simulink model "TLC"  (R2022b)
settings: configuration reference "ERT" (kept outside this file)
undefined symbols (not defined in the file): EGM, FID, IdcMin_P, kiIdcMax_P, kiIdcMin_P, kpIdcMax_P, kpIdcMin_P, OmMechnLimMin_P, pwrIdcMaxDev_P, pwrIdcMinDev_P, SC_fLoLim_C, SC_fUpLim_C, SC_PwrMax_P, SC_TrqMax_P, TQL, trqAddMax_P, trqAddMin_P, Ts_10ms
libraries: simulink x50, MathLib x8, DSMLib x2, slpidlib x1
(part 2 of 2)

== system TLC/TLC_EM/EmOperLim ==
  udclink : Inport
  n : Inport  Port=2
  Abs : Abs  SaturateOnIntegerOverflow=off
  Bus Creator : BusCreator  Inputs=2
  Product : Product
  Product1 : Product
  TrqEmGen_T : Lookup_n-D  DataSpecification=Lookup table object  LookupTableObject=TrqEmGen_T  BreakpointsForDimension1=[250,300,350,400]  BreakpointsForDimension2=[0,500,1000,1500,2000,2500,3000,3500,4000,4500,5000,5500,6000,6500,7000,7500,8000,8500,9000,9500,10000,10500,11000,11500,12000,12500,13000,13500,14000,14500,15000]  BeginIndexSearchUsingPreviousIndexResult=on  Table=reshape([350,350,350,350,350,350,350,350,350,350,350,350,350,350,350,350,350,350,350,350,350,350,350,350,350,350,350,350,350,350,350,350,350,350,350,350,350,350,350,350,350,350,350,350,350,350,350,350,350,350,350,350,350,350,350,350,350,350,350,350,350,350,350,350,350,350,350,350,350,350,350,350,350,350,350,350,350,350,350,350,350,350,350,350,350,350,350,350,350,350,350,350,350,350,350,350,350,350,350,350,350,350,350,350,350,350,350,350,350,350,350,350,350,350,350,350,350,350,350,350,0,0,0,0],4,31)  ExtrapMethod=Clip  UseLastTableValue=on  InternalRulePriority=Speed  OutDataTypeStr=Inherit: Inherit from 'Table data'  RndMeth=Simplest
      settings: InputPortMap=u0,u1
  TrqEmMot_T : Lookup_n-D  DataSpecification=Lookup table object  LookupTableObject=TrqEmMot_T  BreakpointsForDimension1=[250,300,350,400]  BreakpointsForDimension2=[0,500,1000,1500,2000,2500,3000,3500,4000,4500,5000,5500,6000,6500,7000,7500,8000,8500,9000,9500,10000,10500,11000,11500,12000,12500,13000,13500,14000,14500,15000]  BeginIndexSearchUsingPreviousIndexResult=on  Table=reshape([350,350,350,350,350,350,350,350,350,350,350,350,350,350,350,350,350,350,350,350,350,350,350,350,350,350,350,350,350,350,350,350,350,350,350,350,350,350,350,350,350,350,350,350,350,350,350,350,350,350,350,350,350,350,350,350,350,350,350,350,350,350,350,350,350,350,350,350,350,350,350,350,350,350,350,350,350,350,350,350,350,350,350,350,350,350,350,350,350,350,350,350,350,350,350,350,350,350,350,350,350,350,350,350,350,350,350,350,350,350,350,350,350,350,350,350,350,350,350,350,0,0,0,0],4,31)  ExtrapMethod=Clip  UseLastTableValue=on  InternalRulePriority=Speed  OutDataTypeStr=Inherit: Inherit from 'Table data'  RndMeth=Simplest
      settings: InputPortMap=u0,u1
  trqMax : Constant  Value=SC_TrqMax_P  OutDataTypeStr=single
  OperLim : Outport  VectorParamsAs1DForOutWhenUnconnected=off
  wires:
  n/1 -> Abs/1
  Abs/1 -> TrqEmGen_T/2, TrqEmMot_T/2
  TrqEmMot_T/1 -> Product/1
  TrqEmGen_T/1 -> Product1/2
  udclink/1 -> TrqEmGen_T/1, TrqEmMot_T/1
  Bus Creator/1 -> OperLim/1
  Product1/1 -> Bus Creator/2  "trqGenOperLim"
  Product/1 -> Bus Creator/1  "trqMotOperLim"
  trqMax/1 -> Product1/1, Product/2

== system TLC/TLC_EM/IdcLimit ==
  In1 : Inport
  Bus Creator : BusCreator  Inputs=3
  Compare To Constant : simulink/Logic and Bit Operations/Compare To Constant  relop=<  const=1  OutDataTypeStr=boolean
  GLB_PwrMax_P : Constant  Value=SC_TrqMax_P  OutDataTypeStr=single
  Product : Product
  Unary Minus3 : UnaryMinus
  trqGenMotIdcLnkLim_T : Lookup_n-D  NumberOfTableDimensions=1  DataSpecification=Lookup table object  LookupTableObject=trqGenMotIdcLnkLim_T  BreakpointsForDimension1=[-3500 -3000 0 7000 7200]  BeginIndexSearchUsingPreviousIndexResult=on  Table=[0 1 1 1 0]  ExtrapMethod=Clip  UseLastTableValue=on  InternalRulePriority=Speed  OutDataTypeStr=Inherit: Inherit from 'Table data'  RndMeth=Simplest
  IdcLnkLim : Outport  VectorParamsAs1DForOutWhenUnconnected=off
  wires:
  In1/1 -> trqGenMotIdcLnkLim_T/1
  Unary Minus3/1 -> Bus Creator/2  "trqGenIdcLinkLim"
  trqGenMotIdcLnkLim_T/1 -> Compare To Constant/1, Product/2
  Compare To Constant/1 -> Bus Creator/3  "bTrqnLimActv"
  Bus Creator/1 -> IdcLnkLim/1
  GLB_PwrMax_P/1 -> Product/1
  Product/1 -> Bus Creator/1, Unary Minus3/1  "trqMotIdcLinkLim"

== system TLC/TLC_EM/TempClntLim ==
  TempInv : Inport
  Bus Creator : BusCreator  Inputs=3
  GLB_TrqMax_P2 : Constant  Value=SC_TrqMax_P  OutDataTypeStr=single
  Logical Operator : Logic  Operator=OR  AllPortsSameDT=off  OutDataTypeStr=boolean
  Product : Product
  Product1 : Product
  Relational Operator : RelationalOperator  OutDataTypeStr=boolean  RndMeth=Simplest  InputSameDT=off
  Relational Operator1 : RelationalOperator  OutDataTypeStr=boolean  RndMeth=Simplest  InputSameDT=off
  Unary Minus : UnaryMinus
  trqGenTInvLim_T : Lookup_n-D  NumberOfTableDimensions=1  DataSpecification=Lookup table object  LookupTableObject=trqGenTClntLim_T  BreakpointsForDimension1=[100 125 135]  BeginIndexSearchUsingPreviousIndexResult=on  Table=[1 0.8 0]  ExtrapMethod=Clip  UseLastTableValue=on  InternalRulePriority=Speed  OutDataTypeStr=Inherit: Inherit from 'Table data'  RndMeth=Simplest
  trqMotTInvLim_T : Lookup_n-D  NumberOfTableDimensions=1  DataSpecification=Lookup table object  LookupTableObject=trqMotTClntLim_T  BreakpointsForDimension1=[100 125 135]  BeginIndexSearchUsingPreviousIndexResult=on  Table=[1 0.8 0]  ExtrapMethod=Clip  UseLastTableValue=on  InternalRulePriority=Speed  OutDataTypeStr=Inherit: Inherit from 'Table data'  RndMeth=Simplest
  TClntLim : Outport  VectorParamsAs1DForOutWhenUnconnected=off
  wires:
  Product1/1 -> Unary Minus/1, Relational Operator1/2
  trqGenTInvLim_T/1 -> Product1/2
  Unary Minus/1 -> Bus Creator/2  "trqGenTClntLim"
  Bus Creator/1 -> TClntLim/1
  trqMotTInvLim_T/1 -> Product/2
  TempInv/1 -> trqGenTInvLim_T/1, trqMotTInvLim_T/1
  Product/1 -> Bus Creator/1, Relational Operator/2  "trqMotTClntLim"
  GLB_TrqMax_P2/1 -> Relational Operator1/1, Relational Operator/1, Product1/1, Product/1
  Relational Operator/1 -> Logical Operator/1  "bTrqMotTClntLimActv"
  Relational Operator1/1 -> Logical Operator/2  "bTrqGenTClntLimActv"
  Logical Operator/1 -> Bus Creator/3  "bTrqTClntLimActv"

== system TLC/TLC_EM/TempInvLim ==
  TempInv : Inport
  Bus Creator : BusCreator  Inputs=3
  GLB_TrqMax_P2 : Constant  Value=SC_TrqMax_P  OutDataTypeStr=single
  Logical Operator : Logic  Operator=OR  AllPortsSameDT=off  OutDataTypeStr=boolean
  Product : Product
  Product1 : Product
  Relational Operator : RelationalOperator  OutDataTypeStr=boolean  RndMeth=Simplest  InputSameDT=off
  Relational Operator1 : RelationalOperator  OutDataTypeStr=boolean  RndMeth=Simplest  InputSameDT=off
  Unary Minus : UnaryMinus
  trqGenTInvLim_T : Lookup_n-D  NumberOfTableDimensions=1  DataSpecification=Lookup table object  LookupTableObject=trqGenTInvLim_T  BreakpointsForDimension1=[100 125 135]  BeginIndexSearchUsingPreviousIndexResult=on  Table=[1 0.8 0]  ExtrapMethod=Clip  UseLastTableValue=on  InternalRulePriority=Speed  OutDataTypeStr=Inherit: Inherit from 'Table data'  RndMeth=Simplest
  trqMotTInvLim_T : Lookup_n-D  NumberOfTableDimensions=1  DataSpecification=Lookup table object  LookupTableObject=trqMotTInvLim_T  BreakpointsForDimension1=[100 125 135]  BeginIndexSearchUsingPreviousIndexResult=on  Table=[1 0.8 0]  ExtrapMethod=Clip  UseLastTableValue=on  InternalRulePriority=Speed  OutDataTypeStr=Inherit: Inherit from 'Table data'  RndMeth=Simplest
  TInvLim : Outport  VectorParamsAs1DForOutWhenUnconnected=off
  wires:
  Product1/1 -> Unary Minus/1, Relational Operator1/2
  trqGenTInvLim_T/1 -> Product1/2
  Unary Minus/1 -> Bus Creator/2  "trqGenTInvLim"
  Bus Creator/1 -> TInvLim/1
  trqMotTInvLim_T/1 -> Product/2
  TempInv/1 -> trqGenTInvLim_T/1, trqMotTInvLim_T/1
  Product/1 -> Bus Creator/1, Relational Operator/2  "trqMotTInvLim"
  GLB_TrqMax_P2/1 -> Relational Operator1/1, Relational Operator/1, Product1/1, Product/1
  Relational Operator/1 -> Logical Operator/1  "bTrqMotTInvLimActv"
  Relational Operator1/1 -> Logical Operator/2  "bTrqGenTInvLimActv"
  Logical Operator/1 -> Bus Creator/3  "bTrqTinvLimActv"

== system TLC/TLC_EM/TempRtrLim ==
  note: <TODO, change the FID identifier>
  TempRtr : Inport
  Bus Creator1 : BusCreator  Inputs=7
  Bus Creator2 : BusCreator  Inputs=7
  Disable : Subsystem  TreatAsAtomicUnit=on
  Enable : Subsystem  TreatAsAtomicUnit=on
  Enumerated Constant1 : simulink/Sources/Enumerated Constant  OutDataTypeStr=Enum: FID  Value=FID.ReqStandby  SampleTime=inf
      settings: AttributesFormatString=|
      | -------------------------------
      | Enable limitor according to status temperature
  Switch : Switch  Criteria=u2 > Threshold  SaturateOnIntegerOverflow=off  InputSameDT=off
  getFIdSim : DSMLib/getFIdSim  SystemSampleTime=-1  VariantActivationTime=update diagram  Latency=0  AutoFrameSizeCalculation=off
  TRtrLim : Outport  VectorParamsAs1DForOutWhenUnconnected=off
  wires:
  TempRtr/1 -> Disable/1(TmpRtr), Enable/1(TmpRtr)
  Switch/1 -> TRtrLim/1
  Disable/1(pwrMotTRtrLim) -> Bus Creator1/1
  Disable/2(pwrGenTRtrLim) -> Bus Creator1/2
  Disable/3(trqMotTRtrLim) -> Bus Creator1/3
  Disable/4(trqGenTRtrLim) -> Bus Creator1/4
  Disable/5(bTRtrLimActv) -> Bus Creator1/5
  Disable/6(bTrqMotTRtrLimDfcAcive) -> Bus Creator1/6
  Disable/7(bTrqGenTRtrLimDfcAcive) -> Bus Creator1/7
  Enable/1(pwrMotTRtrLim) -> Bus Creator2/1
  Enable/2(pwrGenTRtrLim) -> Bus Creator2/2
  Enable/3(trqMotTRtrLim) -> Bus Creator2/3
  Enable/4(trqGenTRtrLim) -> Bus Creator2/4
  Enable/5(bTRtrLimActv) -> Bus Creator2/5
  Enable/6(bTrqMotTRtrLimDfcAcive) -> Bus Creator2/6
  Enable/7(bTrqGenTRtrLimDfcAcive) -> Bus Creator2/7
  Bus Creator2/1 -> Switch/1
  Bus Creator1/1 -> Switch/3
  Enumerated Constant1/1 -> getFIdSim/1
  getFIdSim/1 -> Switch/2

== system TLC/TLC_EM/TempStrLim ==
  TempStr : Inport
  Bus Creator : BusCreator  Inputs=7
  Enumerated Constant2 : simulink/Sources/Enumerated Constant  OutDataTypeStr=Enum: FID  Value=FID.ReqStandby  SampleTime=inf
      settings: AttributesFormatString=|
      | -------------------------------
      | Enable limitor according to status temperature
  If : If  IfExpression=u1
  If Action Subsystem : Subsystem  TreatAsAtomicUnit=on
  If Action Subsystem1 : Subsystem  TreatAsAtomicUnit=on
  Merge{,1..6} (7 alike) : Merge  InitialOutput=false
  getFIdSim : DSMLib/getFIdSim  SystemSampleTime=-1  VariantActivationTime=update diagram  Latency=0  AutoFrameSizeCalculation=off
  TStrLim : Outport  VectorParamsAs1DForOutWhenUnconnected=off
  wires:
  If/1 -> If Action Subsystem/Action
  If/2 -> If Action Subsystem1/Action
  TempStr/1 -> If Action Subsystem1/1(TmpStr), If Action Subsystem/1(TmpStr)
  If Action Subsystem/1(pwrMotTstrLim) -> Merge/1
  If Action Subsystem/2(pwrGenTstrLim) -> Merge1/1
  If Action Subsystem/7(bTrqGenTstrLimDfcAcive) -> Merge6/1
  If Action Subsystem/6(bTrqMotTstrLimDfcAcive) -> Merge5/1
  If Action Subsystem/5(bTstrLimActv) -> Merge4/1
  If Action Subsystem/4(trqGenTstrLim) -> Merge3/1
  If Action Subsystem/3(trqMotTstrLim) -> Merge2/1
  If Action Subsystem1/1(pwrMotTstrLim) -> Merge/2
  If Action Subsystem1/2(pwrGenTstrLim) -> Merge1/2
  If Action Subsystem1/3(trqMotTstrLim) -> Merge2/2
  If Action Subsystem1/4(trqGenTstrLim) -> Merge3/2
  If Action Subsystem1/5(bTstrLimActv) -> Merge4/2
  If Action Subsystem1/6(bTrqMotTstrLimDfcAcive) -> Merge5/2
  If Action Subsystem1/7(bTrqGenTstrLimDfcAcive) -> Merge6/2
  Merge/1 -> Bus Creator/1  "pwrMotTstrLim"
  Merge1/1 -> Bus Creator/2  "pwrGenTstrLim"
  Merge2/1 -> Bus Creator/3  "trqMotTstrLim"
  Merge3/1 -> Bus Creator/4  "trqGenTstrLim"
  Merge4/1 -> Bus Creator/5  "bTstrLimActv"
  Merge5/1 -> Bus Creator/6  "bTrqMotTstrLimDfcAcive"
  Merge6/1 -> Bus Creator/7  "bTrqGenTstrLimDfcAcive"
  Bus Creator/1 -> TStrLim/1
  Enumerated Constant2/1 -> getFIdSim/1
  getFIdSim/1 -> If/1

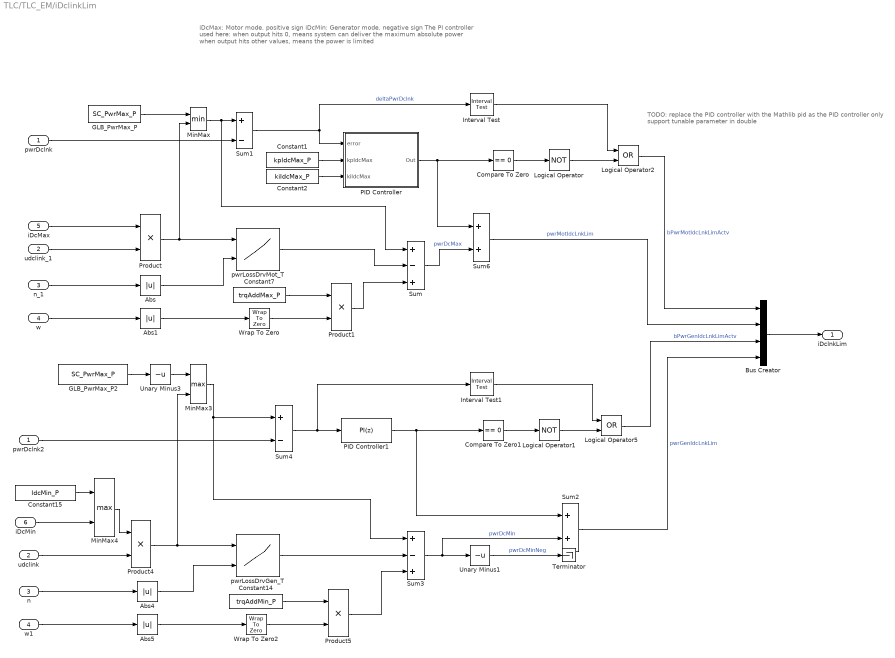
== system TLC/TLC_EM/iDclinkLim ==
  note: TODO:
      | replace the PID controller with the Mathlib pid as the PID controller only support
      | tunable parameter in double
  note: iDcMax: Motor mode. positive sign
      | iDcMin: Generator mode. negative sign
      | The PI controller used here:
      | when output hits 0, means system can deliver the maximum absolute power
      | when output hits other values, means the power is limited
  pwrDclnk : Inport
  udclink : Inport  Port=2
  n : Inport  Port=3
  w : Inport  Port=4
  iDcMax : Inport  Port=5
  iDcMin : Inport  Port=6
  Abs{,1,4..5} (4 alike) : Abs  SaturateOnIntegerOverflow=off
  Bus Creator : BusCreator  Inputs=4
  Compare To Zero : simulink/Logic and Bit Operations/Compare To Zero  relop===  OutDataTypeStr=boolean
  Compare To Zero1 : simulink/Logic and Bit Operations/Compare To Zero  relop===  OutDataTypeStr=boolean
  Constant1 : Constant  Value=kpIdcMax_P
  Constant14 : Constant  Value=trqAddMin_P
  Constant15 : Constant  Value=IdcMin_P
  Constant2 : Constant  Value=kiIdcMax_P
  Constant7 : Constant  Value=trqAddMax_P
  GLB_PwrMax_P : Constant  Value=SC_PwrMax_P  OutDataTypeStr=single
  GLB_PwrMax_P2 : Constant  Value=SC_PwrMax_P  OutDataTypeStr=single
  Interval Test : simulink/Logic and Bit Operations/Interval Test  IntervalClosedRight=on  uplimit=pwrIdcMaxDev_P  IntervalClosedLeft=on  lowlimit=0  OutDataTypeStr=boolean
  Interval Test1 : simulink/Logic and Bit Operations/Interval Test  IntervalClosedRight=on  uplimit=0  IntervalClosedLeft=on  lowlimit=pwrIdcMinDev_P  OutDataTypeStr=boolean
  Logical Operator : Logic  Operator=NOT  AllPortsSameDT=off  OutDataTypeStr=boolean
  Logical Operator1 : Logic  Operator=NOT  AllPortsSameDT=off  OutDataTypeStr=boolean
  Logical Operator2 : Logic  Operator=OR  AllPortsSameDT=off  OutDataTypeStr=boolean
  Logical Operator5 : Logic  Operator=OR  AllPortsSameDT=off  OutDataTypeStr=boolean
  MinMax : MinMax  Inputs=2  InputSameDT=on  SaturateOnIntegerOverflow=on
  MinMax3 : MinMax  Function=max  Inputs=2  InputSameDT=on  SaturateOnIntegerOverflow=on
  MinMax4 : MinMax  Function=max  Inputs=2  InputSameDT=on  SaturateOnIntegerOverflow=on
  PID Controller : MATLAB Function
  PID Controller1 : slpidlib/PID Controller  Controller=PI  Form=Parallel  TimeDomain=Discrete-time  UseExternalTs=off  SampleTime=-1  IntegratorMethod=Forward Euler  FilterMethod=Forward Euler  ControllerParametersSource=internal  P=kpIdcMin_P  I=kiIdcMin_P  UseKiTs=off  D=0  N=100  UseFilter=on  TunerSelectOption=Transfer Function Based (PID Tuner App)  InitialConditionSource=internal  InitialConditionForIntegrator=0  InitialConditionForFilter=0  DifferentiatorICPrevScaledInput=0  ExternalReset=none  TrackingMode=off  Kt=1  LimitOutput=on  SatLimitsSource=internal  UpperSaturationLimit=SC_PwrMax_P  LowerSaturationLimit=0  LinearizeAsGain=on  AntiWindupMode=none  Kb=1  LimitIntegrator=off  UpperIntegratorSaturationLimit=inf  LowerIntegratorSaturationLimit=-inf  POutMin=[]  POutMax=[]  IOutMin=[]  IOutMax=[]  DOutMin=[]  DOutMax=[]  NOutMin=[]  NOutMax=[]  SumOutMin=[]  SumOutMax=[]  SaturationOutMin=[]  SaturationOutMax=[]  PParamMin=[]  PParamMax=[]  IParamMin=[]  IParamMax=[]  DParamMin=[]  DParamMax=[]  NParamMin=[]  NParamMax=[]  KbParamMin=[]  KbParamMax=[]  KtParamMin=[]  KtParamMax=[]  KbOutMin=[]  KbOutMax=[]  KtOutMin=[]  KtOutMax=[]  IntegratorOutMin=[]  IntegratorOutMax=[]  FilterOutMin=[]  FilterOutMax=[]  SumI1OutMin=[]  SumI1OutMax=[]  SumI2OutMin=[]  SumI2OutMax=[]  SumI3OutMin=[]  SumI3OutMax=[]  SumI4OutMin=[]  SumI4OutMax=[]  SumDOutMin=[]  SumDOutMax=[]  DifferentiatorOutMin=[]  DifferentiatorOutMax=[]  FilterDiffOutCoefMin=[]  FilterDiffOutCoefMax=[]  ReciprocalOutMin=[]  ReciprocalOutMax=[]  SumDenOutMin=[]  SumDenOutMax=[]  SumNumOutMin=[]  SumNumOutMax=[]  DivideOutMin=[]  DivideOutMax=[]  UdiffTsProdOutMin=[]  UdiffTsProdOutMax=[]  NTsProdOutMin=[]  NTsProdOutMax=[]  UintegralTsProdOutMin=[]  UintegralTsProdOutMax=[]  UngainTsProdOutMin=[]  UngainTsProdOutMax=[]  ClampingZeroOutDataTypeStr=Inherit: Inherit via back propagation  ClampingZeroOutMin=[]  ClampingZeroOutMax=[]  FilterDenConstantOutDataTypeStr=Inherit: Inherit via back propagation  FilterDenConstantOutMin=[]  FilterDenConstantOutMax=[]  PCopyOutDataTypeStr=Inherit: Inherit via back propagation  PCopyOutMin=[]  PCopyOutMax=[]  NCopyOutDataTypeStr=Inherit: Inherit via back propagation  NCopyOutMin=[]  NCopyOutMax=[]  IntegratorContinuousStateAttributes=''  IntegratorStateMustResolveToSignalObject=off  IntegratorRTWStateStorageClass=Auto  FilterContinuousStateAttributes=''  FilterStateMustResolveToSignalObject=off  FilterRTWStateStorageClass=Auto  ParallelPVariant=InternalParameters  IdealPVariant=Disabled  IVariant=InternalParameters  DVariant=Disabled  IntegratorVariant=Discrete  SatVariant=Enabled  AWVariant=Passthrough  PCopyVariant=Disabled  TRVariant=Disabled  FdbkBlocksVariant=Forward  IdealPFdbkVariant=Disabled  SatFdbkVariant=Disabled  DerivativeFilterVariant=Disabled  NVariant=Disabled  NCopyVariant=Disabled_SignalSpec  FilterICVariant=Disabled  IntegratorICVariant=InternalICs  ExternalResetVariant=Disabled  TRSumVariant=Passthrough  SumFdbkVariant=Disabled  SumVariant=Sum_PI  TsampFilterVariant=InternalTs  TsampNgainVariant=Passthrough  TsampIntegralVariant=Passthrough  ExternalSaturationOutDataTypeStr=Inherit: Same as second input
  Product{,1,4..5} (4 alike) : Product
  Sum : Sum  Inputs=+-+  InputSameDT=on  SaturateOnIntegerOverflow=on  OutDataTypeStr=Inherit: Same as first input
  Sum1 : Sum  Inputs=+-  InputSameDT=on  SaturateOnIntegerOverflow=on  OutDataTypeStr=Inherit: Same as first input
  Sum2 : Sum  InputSameDT=on  SaturateOnIntegerOverflow=on  OutDataTypeStr=Inherit: Same as first input
  Sum3 : Sum  Inputs=+-+  InputSameDT=on  SaturateOnIntegerOverflow=on  OutDataTypeStr=Inherit: Same as first input
  Sum4 : Sum  Inputs=+-  InputSameDT=on  SaturateOnIntegerOverflow=on  OutDataTypeStr=Inherit: Same as first input
  Sum6 : Sum  InputSameDT=on  SaturateOnIntegerOverflow=on  OutDataTypeStr=Inherit: Same as first input
  Terminator : Terminator
  Unary Minus1 : UnaryMinus
  Unary Minus3 : UnaryMinus
  Wrap To Zero : simulink/Discontinuities/Wrap To Zero  Threshold=OmMechnLimMin_P
  Wrap To Zero2 : simulink/Discontinuities/Wrap To Zero  Threshold=OmMechnLimMin_P
  n_1 : InportShadow  Port=3
  pwrDclnk2 : InportShadow
  pwrLossDrvGen_T : Lookup_n-D  DataSpecification=Lookup table object  LookupTableObject=pwrLossDrvGen_T  BreakpointsForDimension1=|  BreakpointsForDimension2=|  BeginIndexSearchUsingPreviousIndexResult=on  Table=|  ExtrapMethod=Clip  UseLastTableValue=on  InternalRulePriority=Speed  OutDataTypeStr=Inherit: Inherit from 'Table data'  InputSameDT=off
      BreakpointsForDimension1=|
      | [0
      | 0.1
      | 0.2
      | 0.3
      | 0.4
      | 0.5
      | 0.6
      | 0.7
      | 0.8
      | 0.9
      | 0.94
      | 0.98
      | 1
      | 1.16]
      Table=|
      | reshape([500 	500 	500 	500 	500 	500 	500 	500 	500 	500 	500 
      | 500 	500 	500 	500 	500 	499 	489 	481 	476 	471 	468 
      | 412 	412 	328 	300 	286 	277 	272 	267 	264 	262 	260 
      | 297 	297 	240 	221 	212 	206 	202 	199 	197 	196 	195 
      | 245 	245 	201 	187 	179 	175 	172 	170 	169 	167 	166 
      | 219 	219 	183 	172 	166 	162 	160 	158 	157 	156 	155 
      | 184 	184 	157 	149 	144 	141 	140 	138 	137 	137 	136 
      | 156 	156 	137 	130 	127 	125 	124 	123 	122 	122 	121 
      | 134 	134 	120 	115 	113 	112 	111 	110 	110 	109 	109 
      | 116 	116 	106 	103 	102 	101 	100 	100 	100 	100 	100 
      | 109 	109 	101 	100 	100 	100 	100 	100 	100 	100 	100 
      | 103 	103 	100 	100 	100 	100 	100 	100 	100 	100 	100 
      | 100 	100 	100 	100 	100 	100 	100 	100 	100 	100 	100 
      | 100 	100 	100 	100 	100 	100 	100 	100 	100 	100 	100 ],14,11)
      BreakpointsForDimension2=|
      | [0	50	100	150	200	250	300	350	400	450	500
      | ]
      settings: InputPortMap=u0,u1
  pwrLossDrvMot_T : Lookup_n-D  DataSpecification=Lookup table object  LookupTableObject=pwrLossDrvMot_T  BreakpointsForDimension1=|  BreakpointsForDimension2=|  BeginIndexSearchUsingPreviousIndexResult=on  Table=|  ExtrapMethod=Clip  UseLastTableValue=on  InternalRulePriority=Speed  OutDataTypeStr=Inherit: Inherit from 'Table data'  InputSameDT=off
      BreakpointsForDimension1=|
      | [0
      | 0.1
      | 0.2
      | 0.3
      | 0.4
      | 0.5
      | 0.6
      | 0.7
      | 0.8
      | 0.9
      | 0.94
      | 0.98
      | 1
      | 1.16]
      Table=|
      | reshape([500 	500 	500 	500 	500 	500 	500 	500 	500 	500 	500 
      | 500 	500 	500 	500 	500 	499 	489 	481 	476 	471 	468 
      | 412 	412 	328 	300 	286 	277 	272 	267 	264 	262 	260 
      | 297 	297 	240 	221 	212 	206 	202 	199 	197 	196 	195 
      | 245 	245 	201 	187 	179 	175 	172 	170 	169 	167 	166 
      | 219 	219 	183 	172 	166 	162 	160 	158 	157 	156 	155 
      | 184 	184 	157 	149 	144 	141 	140 	138 	137 	137 	136 
      | 156 	156 	137 	130 	127 	125 	124 	123 	122 	122 	121 
      | 134 	134 	120 	115 	113 	112 	111 	110 	110 	109 	109 
      | 116 	116 	106 	103 	102 	101 	100 	100 	100 	100 	100 
      | 109 	109 	101 	100 	100 	100 	100 	100 	100 	100 	100 
      | 103 	103 	100 	100 	100 	100 	100 	100 	100 	100 	100 
      | 100 	100 	100 	100 	100 	100 	100 	100 	100 	100 	100 
      | 100 	100 	100 	100 	100 	100 	100 	100 	100 	100 	100 ],14,11)
      BreakpointsForDimension2=|
      | [0	50	100	150	200	250	300	350	400	450	500
      | ]
      settings: InputPortMap=u0,u1
  udclink_1 : InportShadow  Port=2
  w1 : InportShadow  Port=4
  iDclnkLim : Outport  VectorParamsAs1DForOutWhenUnconnected=off
  wires:
  Constant7/1 -> Product1/1
  Sum1/1 -> PID Controller/1(error), Interval Test/1  "deltaPwrDclnk"
  Logical Operator2/1 -> Bus Creator/1  "bPwrMotIdcLnkLimActv"
  Logical Operator/1 -> Logical Operator2/2
  pwrDclnk/1 -> Sum1/2
  w1/1 -> Abs5/1
  MinMax3/1 -> Sum3/1, Sum4/1
  Sum3/1 -> Unary Minus1/1, Sum2/2  "pwrDcMin"
  Sum6/1 -> Bus Creator/2  "pwrMotIdcLnkLim"
  pwrDclnk2/1 -> Sum4/2
  Product4/1 -> pwrLossDrvGen_T/1, MinMax3/2
  Logical Operator5/1 -> Bus Creator/3  "bPwrGenIdcLnkLimActv"
  GLB_PwrMax_P2/1 -> Unary Minus3/1
  Product5/1 -> Sum3/3
  Wrap To Zero2/1 -> Product5/2
  Sum2/1 -> Bus Creator/4  "pwrGenIdcLnkLim"
  Constant14/1 -> Product5/1
  udclink/1 -> Product4/2
  Product1/1 -> Sum/3
  pwrLossDrvGen_T/1 -> Sum3/2
  Abs5/1 -> Wrap To Zero2/1
  n/1 -> Abs4/1
  Interval Test1/1 -> Logical Operator5/1
  Unary Minus3/1 -> MinMax3/1
  w/1 -> Abs1/1
  Abs1/1 -> Wrap To Zero/1
  Sum/1 -> Sum6/2  "pwrDcMax"
  iDcMax/1 -> Product/1
  udclink_1/1 -> Product/2
  GLB_PwrMax_P/1 -> MinMax/1
  Product/1 -> pwrLossDrvMot_T/1, MinMax/2
  n_1/1 -> Abs/1
  MinMax/1 -> Sum/1, Sum1/1
  Abs/1 -> pwrLossDrvMot_T/2
  pwrLossDrvMot_T/1 -> Sum/2
  Compare To Zero/1 -> Logical Operator/1
  Interval Test/1 -> Logical Operator2/1
  Constant15/1 -> MinMax4/1
  Wrap To Zero/1 -> Product1/2
  MinMax4/1 -> Product4/1
  iDcMin/1 -> MinMax4/2
  Bus Creator/1 -> iDclnkLim/1
  PID Controller/1(Out) -> Sum6/1, Compare To Zero/1
  Sum4/1 -> Interval Test1/1, PID Controller1/1
  Compare To Zero1/1 -> Logical Operator1/1
  PID Controller1/1 -> Compare To Zero1/1, Sum2/1
  Logical Operator1/1 -> Logical Operator5/2
  Unary Minus1/1 -> Terminator/1  "pwrDcMinNeg"
  Abs4/1 -> pwrLossDrvGen_T/2
  Constant1/1 -> PID Controller/2(kpIdcMax)
  Constant2/1 -> PID Controller/3(kiIdcMax)

== system TLC/TLC_EM/nLimit ==
  In1 : Inport
  Bus Creator : BusCreator  Inputs=3
  Compare To Constant : simulink/Logic and Bit Operations/Compare To Constant  relop=<  const=1  OutDataTypeStr=boolean
  GLB_PwrMax_P : Constant  Value=SC_TrqMax_P  OutDataTypeStr=single
  Product : Product
  Unary Minus3 : UnaryMinus
  pwrGenMotnLim_T : Lookup_n-D  NumberOfTableDimensions=1  DataSpecification=Lookup table object  LookupTableObject=pwrGenMotnLim_T  BreakpointsForDimension1=[-3500 -3000 0 7000 7200]  BeginIndexSearchUsingPreviousIndexResult=on  Table=[0 1 1 1 0]  ExtrapMethod=Clip  UseLastTableValue=on  InternalRulePriority=Speed  OutDataTypeStr=Inherit: Inherit from 'Table data'  RndMeth=Simplest
  Out1 : Outport  VectorParamsAs1DForOutWhenUnconnected=off
  wires:
  In1/1 -> pwrGenMotnLim_T/1
  Unary Minus3/1 -> Bus Creator/2  "trqGennLim"
  pwrGenMotnLim_T/1 -> Compare To Constant/1, Product/2
  Compare To Constant/1 -> Bus Creator/3  "bTrqnLimActv"
  Bus Creator/1 -> Out1/1
  GLB_PwrMax_P/1 -> Product/1
  Product/1 -> Bus Creator/1, Unary Minus3/1  "trqMotnLim"

== system TLC/TLC_EM/ratIsHeatPntLimit ==
  ratIsHeatPnt : Inport
  Bus Creator : BusCreator  Inputs=3
  Compare To Constant : simulink/Logic and Bit Operations/Compare To Constant  relop=<  const=1  OutDataTypeStr=boolean
  Display : Display
  GLB_PwrMax_P : Constant  Value=SC_TrqMax_P  OutDataTypeStr=single
  Product : Product
  Unary Minus3 : UnaryMinus
  ratIsHeatPntLim_T : Lookup_n-D  NumberOfTableDimensions=1  DataSpecification=Lookup table object  LookupTableObject=ratIsHeatPntLim_T  BreakpointsForDimension1=[-3500 -3000 0 7000 7200]  BeginIndexSearchUsingPreviousIndexResult=on  Table=[0 1 1 1 0]  ExtrapMethod=Clip  UseLastTableValue=on  InternalRulePriority=Speed  OutDataTypeStr=Inherit: Inherit from 'Table data'  RndMeth=Simplest
  ratIsHeatPntLimit : Outport  VectorParamsAs1DForOutWhenUnconnected=off
  wires:
  Product/1 -> Unary Minus3/1, Bus Creator/1  "ratIsHeatPntMotLim"
  GLB_PwrMax_P/1 -> Product/1
  Bus Creator/1 -> ratIsHeatPntLimit/1
  Compare To Constant/1 -> Bus Creator/3  "bRatIsHeatPntActv"
  ratIsHeatPntLim_T/1 -> Product/2, Display/1, Compare To Constant/1
  Unary Minus3/1 -> Bus Creator/2  "ratIsHeatPntGenLim"
  ratIsHeatPnt/1 -> ratIsHeatPntLim_T/1

== system TLC/TLC_EM/uDclinkLim ==
  note: uDcMin: Motor mode.
      | uDcMax: Generator mode.
      | Linear method
  udclink : Inport
  uDcMax : Inport  Port=2
  uDcMin : Inport  Port=3
  Bus Creator : BusCreator  Inputs=4
  Compare To Constant : simulink/Logic and Bit Operations/Compare To Constant  relop=<  const=1  OutDataTypeStr=boolean
  Compare To Constant1 : simulink/Logic and Bit Operations/Compare To Constant  relop=<  const=1  OutDataTypeStr=boolean
  GLB_PwrMax_P : Constant  Value=SC_PwrMax_P  OutDataTypeStr=single
  Product : Product
  Product1 : Product
  Sum5 : Sum  Inputs=+-  InputSameDT=on  SaturateOnIntegerOverflow=on  OutDataTypeStr=Inherit: Same as first input
  Sum7 : Sum  Inputs=+-  InputSameDT=on  SaturateOnIntegerOverflow=on  OutDataTypeStr=Inherit: Same as first input
  pwrGenUdclnkLim_T : Lookup_n-D  NumberOfTableDimensions=1  DataSpecification=Lookup table object  LookupTableObject=pwrGenUdclnkLim_T  BreakpointsForDimension1=[-8 -4 -2 0 5 6 7 8]  BeginIndexSearchUsingPreviousIndexResult=on  Table=[1 0.4 0.3 0 0 0 0 0]  ExtrapMethod=Clip  UseLastTableValue=on  InternalRulePriority=Speed  OutDataTypeStr=Inherit: Inherit from 'Table data'  RndMeth=Simplest
  pwrMotUdclnkLim_T : Lookup_n-D  NumberOfTableDimensions=1  DataSpecification=Lookup table object  LookupTableObject=pwrMotUdclnkLim_T  BreakpointsForDimension1=[-13 -11 -2 -1 0 1 2 5]  BeginIndexSearchUsingPreviousIndexResult=on  Table=[0 0 0 0.1 0.2 0.3 0.5 1]  ExtrapMethod=Clip  UseLastTableValue=on  InternalRulePriority=Speed  OutDataTypeStr=Inherit: Inherit from 'Table data'  RndMeth=Simplest  InputSameDT=off
  iDclnkLim : Outport  VectorParamsAs1DForOutWhenUnconnected=off
  wires:
  Bus Creator/1 -> iDclnkLim/1
  Sum5/1 -> pwrGenUdclnkLim_T/1
  GLB_PwrMax_P/1 -> Product1/1, Product/1
  udclink/1 -> Sum7/1, Sum5/1
  uDcMax/1 -> Sum5/2
  uDcMin/1 -> Sum7/2
  Sum7/1 -> pwrMotUdclnkLim_T/1
  pwrGenUdclnkLim_T/1 -> Compare To Constant/1, Product/2
  pwrMotUdclnkLim_T/1 -> Compare To Constant1/1, Product1/2
  Product/1 -> Bus Creator/1  "pwrGenUdclnkLim"
  Compare To Constant/1 -> Bus Creator/2  "bPwrGenUdclnkLimActv"
  Product1/1 -> Bus Creator/3  "pwrMotUdclnkLim"
  Compare To Constant1/1 -> Bus Creator/4  "bPwrMotUdclnkLimActv"

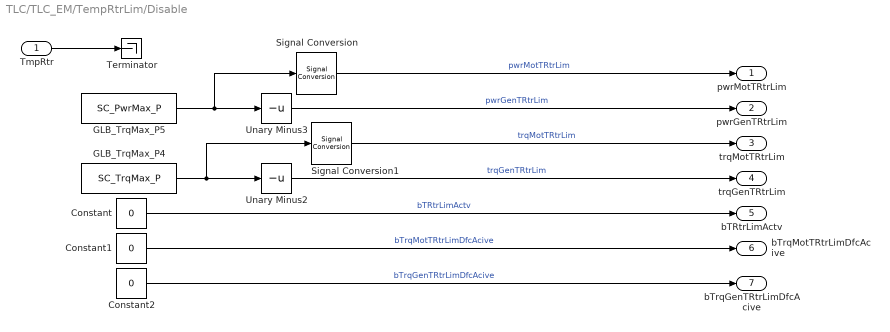
== system TLC/TLC_EM/TempRtrLim/Disable ==
  TmpRtr : Inport
  Constant : Constant  Value=0  OutDataTypeStr=boolean
  Constant1 : Constant  Value=0  OutDataTypeStr=boolean
  Constant2 : Constant  Value=0  OutDataTypeStr=boolean
  GLB_TrqMax_P4 : Constant  Value=SC_TrqMax_P  OutDataTypeStr=single
  GLB_TrqMax_P5 : Constant  Value=SC_PwrMax_P  OutDataTypeStr=single
  Signal Conversion : SignalConversion  OverrideOpt=off
  Signal Conversion1 : SignalConversion  OverrideOpt=off
  Terminator : Terminator
  Unary Minus2 : UnaryMinus
  Unary Minus3 : UnaryMinus
  pwrMotTRtrLim : Outport  VectorParamsAs1DForOutWhenUnconnected=off
  pwrGenTRtrLim : Outport  Port=2  VectorParamsAs1DForOutWhenUnconnected=off
  trqMotTRtrLim : Outport  Port=3  VectorParamsAs1DForOutWhenUnconnected=off
  trqGenTRtrLim : Outport  Port=4  VectorParamsAs1DForOutWhenUnconnected=off
  bTRtrLimActv : Outport  Port=5  VectorParamsAs1DForOutWhenUnconnected=off
  bTrqMotTRtrLimDfcAcive : Outport  Port=6  VectorParamsAs1DForOutWhenUnconnected=off
  bTrqGenTRtrLimDfcAcive : Outport  Port=7  VectorParamsAs1DForOutWhenUnconnected=off
  wires:
  Constant2/1 -> bTrqGenTRtrLimDfcAcive/1  "bTrqGenTRtrLimDfcAcive"
  Constant1/1 -> bTrqMotTRtrLimDfcAcive/1  "bTrqMotTRtrLimDfcAcive"
  Constant/1 -> bTRtrLimActv/1  "bTRtrLimActv"
  TmpRtr/1 -> Terminator/1
  Unary Minus3/1 -> pwrGenTRtrLim/1  "pwrGenTRtrLim"
  Unary Minus2/1 -> trqGenTRtrLim/1  "trqGenTRtrLim"
  GLB_TrqMax_P5/1 -> Signal Conversion/1, Unary Minus3/1
  GLB_TrqMax_P4/1 -> Signal Conversion1/1, Unary Minus2/1
  Signal Conversion/1 -> pwrMotTRtrLim/1  "pwrMotTRtrLim"
  Signal Conversion1/1 -> trqMotTRtrLim/1  "trqMotTRtrLim"

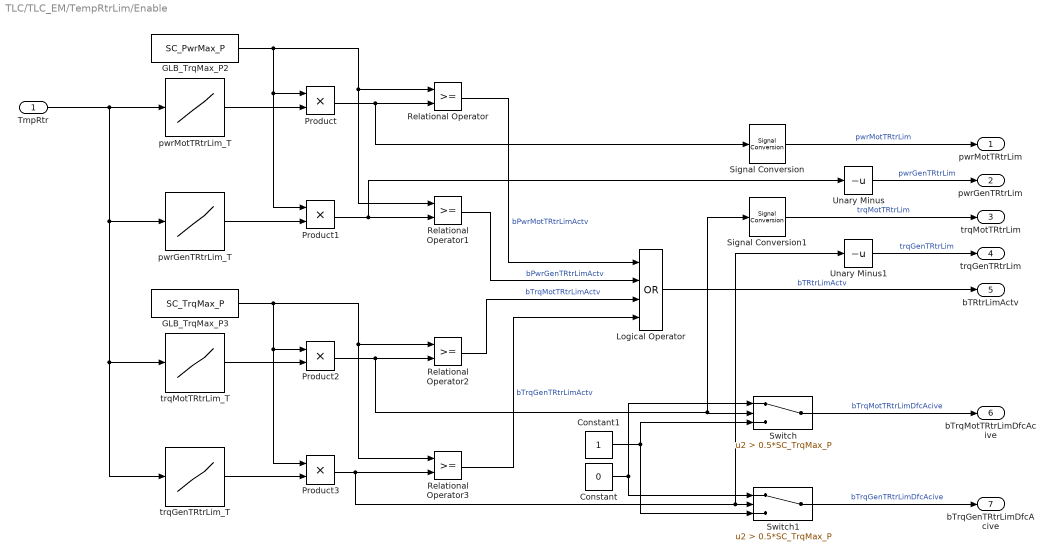
== system TLC/TLC_EM/TempRtrLim/Enable ==
  TmpRtr : Inport
  Constant : Constant  Value=0  OutDataTypeStr=boolean
  Constant1 : Constant  OutDataTypeStr=boolean
  GLB_TrqMax_P2 : Constant  Value=SC_PwrMax_P  OutDataTypeStr=single
  GLB_TrqMax_P3 : Constant  Value=SC_TrqMax_P  OutDataTypeStr=single
  Logical Operator : Logic  Operator=OR  Inputs=4  AllPortsSameDT=off  OutDataTypeStr=boolean
  Product{,1..3} (4 alike) : Product
  Relational Operator{,1..3} (4 alike) : RelationalOperator  OutDataTypeStr=boolean  RndMeth=Simplest  InputSameDT=off
  Signal Conversion : SignalConversion  OverrideOpt=off
  Signal Conversion1 : SignalConversion  OverrideOpt=off
  Switch : Switch  Criteria=u2 > Threshold  Threshold=0.5*SC_TrqMax_P  SaturateOnIntegerOverflow=off  InputSameDT=off
      settings: AttributesFormatString=|
      | ------------------------------
      | x<0.5*GLB_TrqMax_P-->SetDFC true
  Switch1 : Switch  Criteria=u2 > Threshold  Threshold=0.5*SC_TrqMax_P  SaturateOnIntegerOverflow=off  InputSameDT=off
      settings: AttributesFormatString=|
      | ------------------------------
      | x<0.5*GLB_TrqMax_P-->SetDFC true
  Unary Minus : UnaryMinus
  Unary Minus1 : UnaryMinus
  pwrGenTRtrLim_T : Lookup_n-D  NumberOfTableDimensions=1  DataSpecification=Lookup table object  LookupTableObject=pwrGenTRtrLim_T  BreakpointsForDimension1=[140 165]  BeginIndexSearchUsingPreviousIndexResult=on  Table=[1 0.06]  ExtrapMethod=Clip  UseLastTableValue=on  InternalRulePriority=Speed  OutDataTypeStr=Inherit: Inherit from 'Table data'  RndMeth=Simplest
  pwrMotTRtrLim_T : Lookup_n-D  NumberOfTableDimensions=1  DataSpecification=Lookup table object  LookupTableObject=pwrMotTRtrLim_T  BreakpointsForDimension1=[140 165]  BeginIndexSearchUsingPreviousIndexResult=on  Table=[1 0]  ExtrapMethod=Clip  UseLastTableValue=on  InternalRulePriority=Speed  OutDataTypeStr=Inherit: Inherit from 'Table data'  RndMeth=Simplest
  trqGenTRtrLim_T : Lookup_n-D  NumberOfTableDimensions=1  DataSpecification=Lookup table object  LookupTableObject=trqGenTRtrLim_T  BreakpointsForDimension1=[140 165]  BeginIndexSearchUsingPreviousIndexResult=on  Table=[1 0.1]  ExtrapMethod=Clip  UseLastTableValue=on  InternalRulePriority=Speed  OutDataTypeStr=Inherit: Inherit from 'Table data'  RndMeth=Simplest
  trqMotTRtrLim_T : Lookup_n-D  NumberOfTableDimensions=1  DataSpecification=Lookup table object  LookupTableObject=trqMotTRtrLim_T  BreakpointsForDimension1=[140 165]  BeginIndexSearchUsingPreviousIndexResult=on  Table=[1 0]  ExtrapMethod=Clip  UseLastTableValue=on  InternalRulePriority=Speed  OutDataTypeStr=Inherit: Inherit from 'Table data'  RndMeth=Simplest
  pwrMotTRtrLim : Outport  VectorParamsAs1DForOutWhenUnconnected=off
  pwrGenTRtrLim : Outport  Port=2  VectorParamsAs1DForOutWhenUnconnected=off
  trqMotTRtrLim : Outport  Port=3  VectorParamsAs1DForOutWhenUnconnected=off
  trqGenTRtrLim : Outport  Port=4  VectorParamsAs1DForOutWhenUnconnected=off
  bTRtrLimActv : Outport  Port=5  VectorParamsAs1DForOutWhenUnconnected=off
  bTrqMotTRtrLimDfcAcive : Outport  Port=6  VectorParamsAs1DForOutWhenUnconnected=off
  bTrqGenTRtrLimDfcAcive : Outport  Port=7  VectorParamsAs1DForOutWhenUnconnected=off
  wires:
  Product3/1 -> Relational Operator3/2, Unary Minus1/1, Switch1/2
  Switch1/1 -> bTrqGenTRtrLimDfcAcive/1  "bTrqGenTRtrLimDfcAcive"
  Switch/1 -> bTrqMotTRtrLimDfcAcive/1  "bTrqMotTRtrLimDfcAcive"
  Constant1/1 -> Switch/3, Switch1/3
  Constant/1 -> Switch1/1, Switch/1
  Logical Operator/1 -> bTRtrLimActv/1  "bTRtrLimActv"
  Unary Minus1/1 -> trqGenTRtrLim/1  "trqGenTRtrLim"
  Relational Operator3/1 -> Logical Operator/4  "bTrqGenTRtrLimActv"
  Relational Operator2/1 -> Logical Operator/3  "bTrqMotTRtrLimActv"
  Product2/1 -> Signal Conversion1/1, Switch/2, Relational Operator2/2
  GLB_TrqMax_P3/1 -> Relational Operator2/1, Relational Operator3/1, Product2/1, Product3/1
  trqGenTRtrLim_T/1 -> Product3/2
  trqMotTRtrLim_T/1 -> Product2/2
  Unary Minus/1 -> pwrGenTRtrLim/1  "pwrGenTRtrLim"
  Relational Operator1/1 -> Logical Operator/2  "bPwrGenTRtrLimActv"
  Relational Operator/1 -> Logical Operator/1  "bPwrMotTRtrLimActv"
  Product1/1 -> Relational Operator1/2, Unary Minus/1
  Product/1 -> Relational Operator/2, Signal Conversion/1
  GLB_TrqMax_P2/1 -> Product1/1, Product/1, Relational Operator1/1, Relational Operator/1
  pwrGenTRtrLim_T/1 -> Product1/2
  pwrMotTRtrLim_T/1 -> Product/2
  TmpRtr/1 -> pwrMotTRtrLim_T/1, pwrGenTRtrLim_T/1, trqGenTRtrLim_T/1, trqMotTRtrLim_T/1
  Signal Conversion/1 -> pwrMotTRtrLim/1  "pwrMotTRtrLim"
  Signal Conversion1/1 -> trqMotTRtrLim/1  "trqMotTRtrLim"

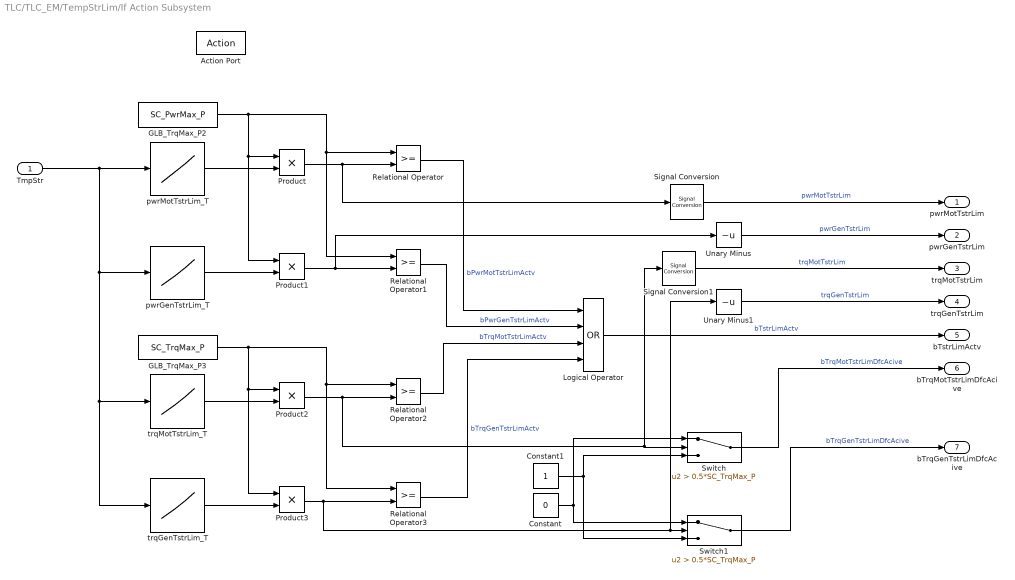
== system TLC/TLC_EM/TempStrLim/If Action Subsystem ==
  TmpStr : Inport
  Action Port : ActionPort  ActionPortLabel=if(u1)
  Constant : Constant  Value=0  OutDataTypeStr=boolean
  Constant1 : Constant  OutDataTypeStr=boolean
  GLB_TrqMax_P2 : Constant  Value=SC_PwrMax_P  OutDataTypeStr=single
  GLB_TrqMax_P3 : Constant  Value=SC_TrqMax_P  OutDataTypeStr=single
  Logical Operator : Logic  Operator=OR  Inputs=4  AllPortsSameDT=off  OutDataTypeStr=boolean
  Product{,1..3} (4 alike) : Product
  Relational Operator{,1..3} (4 alike) : RelationalOperator  OutDataTypeStr=boolean  RndMeth=Simplest  InputSameDT=off
  Signal Conversion : SignalConversion  OverrideOpt=off
  Signal Conversion1 : SignalConversion  OverrideOpt=off
  Switch : Switch  Criteria=u2 > Threshold  Threshold=0.5*SC_TrqMax_P  SaturateOnIntegerOverflow=off  InputSameDT=off
      settings: AttributesFormatString=|
      | ------------------------------
      | x<0.5*GLB_TrqMax_P-->SetDFC true
  Switch1 : Switch  Criteria=u2 > Threshold  Threshold=0.5*SC_TrqMax_P  SaturateOnIntegerOverflow=off  InputSameDT=off
      settings: AttributesFormatString=|
      | ------------------------------
      | x<0.5*GLB_TrqMax_P-->SetDFC true
  Unary Minus : UnaryMinus
  Unary Minus1 : UnaryMinus
  pwrGenTstrLim_T : Lookup_n-D  NumberOfTableDimensions=1  DataSpecification=Lookup table object  LookupTableObject=pwrGenTstrLim_T  BreakpointsForDimension1=[160:10:200]  BeginIndexSearchUsingPreviousIndexResult=on  Table=[1 0.95 0.8 0.2 0 ]  ExtrapMethod=Clip  UseLastTableValue=on  InternalRulePriority=Speed  OutDataTypeStr=Inherit: Inherit from 'Table data'  RndMeth=Simplest
  pwrMotTstrLim_T : Lookup_n-D  NumberOfTableDimensions=1  DataSpecification=Lookup table object  LookupTableObject=pwrMotTstrLim_T  BreakpointsForDimension1=[160:10:200]  BeginIndexSearchUsingPreviousIndexResult=on  Table=[1 0.95 0.8 0.2 0 ]  ExtrapMethod=Clip  UseLastTableValue=on  InternalRulePriority=Speed  OutDataTypeStr=Inherit: Inherit from 'Table data'  RndMeth=Simplest
  trqGenTstrLim_T : Lookup_n-D  NumberOfTableDimensions=1  DataSpecification=Lookup table object  LookupTableObject=trqGenTstrLim_T  BreakpointsForDimension1=[160:10:200]  BeginIndexSearchUsingPreviousIndexResult=on  Table=[1 0.95 0.8 0.2 0 ]  ExtrapMethod=Clip  UseLastTableValue=on  InternalRulePriority=Speed  OutDataTypeStr=Inherit: Inherit from 'Table data'  RndMeth=Simplest
  trqMotTstrLim_T : Lookup_n-D  NumberOfTableDimensions=1  DataSpecification=Lookup table object  LookupTableObject=trqMotTstrLim_T  BreakpointsForDimension1=[160:10:200]  BeginIndexSearchUsingPreviousIndexResult=on  Table=[1 0.95 0.8 0.2 0 ]  ExtrapMethod=Clip  UseLastTableValue=on  InternalRulePriority=Speed  OutDataTypeStr=Inherit: Inherit from 'Table data'  RndMeth=Simplest
  pwrMotTstrLim : Outport  VectorParamsAs1DForOutWhenUnconnected=off
  pwrGenTstrLim : Outport  Port=2  VectorParamsAs1DForOutWhenUnconnected=off
  trqMotTstrLim : Outport  Port=3  VectorParamsAs1DForOutWhenUnconnected=off
  trqGenTstrLim : Outport  Port=4  VectorParamsAs1DForOutWhenUnconnected=off
  bTstrLimActv : Outport  Port=5  VectorParamsAs1DForOutWhenUnconnected=off
  bTrqMotTstrLimDfcAcive : Outport  Port=6  VectorParamsAs1DForOutWhenUnconnected=off
  bTrqGenTstrLimDfcAcive : Outport  Port=7  VectorParamsAs1DForOutWhenUnconnected=off
  wires:
  TmpStr/1 -> trqMotTstrLim_T/1, trqGenTstrLim_T/1, pwrGenTstrLim_T/1, pwrMotTstrLim_T/1
  pwrMotTstrLim_T/1 -> Product/2
  pwrGenTstrLim_T/1 -> Product1/2
  GLB_TrqMax_P2/1 -> Relational Operator/1, Relational Operator1/1, Product/1, Product1/1
  Product/1 -> Signal Conversion/1, Relational Operator/2
  Product1/1 -> Unary Minus/1, Relational Operator1/2
  Relational Operator/1 -> Logical Operator/1  "bPwrMotTstrLimActv"
  Relational Operator1/1 -> Logical Operator/2  "bPwrGenTstrLimActv"
  Unary Minus/1 -> pwrGenTstrLim/1  "pwrGenTstrLim"
  trqMotTstrLim_T/1 -> Product2/2
  trqGenTstrLim_T/1 -> Product3/2
  GLB_TrqMax_P3/1 -> Product3/1, Product2/1, Relational Operator3/1, Relational Operator2/1
  Product2/1 -> Relational Operator2/2, Switch/2, Signal Conversion1/1
  Relational Operator2/1 -> Logical Operator/3  "bTrqMotTstrLimActv"
  Relational Operator3/1 -> Logical Operator/4  "bTrqGenTstrLimActv"
  Unary Minus1/1 -> trqGenTstrLim/1  "trqGenTstrLim"
  Logical Operator/1 -> bTstrLimActv/1  "bTstrLimActv"
  Constant/1 -> Switch/1, Switch1/1
  Constant1/1 -> Switch1/3, Switch/3
  Switch/1 -> bTrqMotTstrLimDfcAcive/1  "bTrqMotTstrLimDfcAcive"
  Switch1/1 -> bTrqGenTstrLimDfcAcive/1  "bTrqGenTstrLimDfcAcive"
  Product3/1 -> Switch1/2, Unary Minus1/1, Relational Operator3/2
  Signal Conversion/1 -> pwrMotTstrLim/1  "pwrMotTstrLim"
  Signal Conversion1/1 -> trqMotTstrLim/1  "trqMotTstrLim"

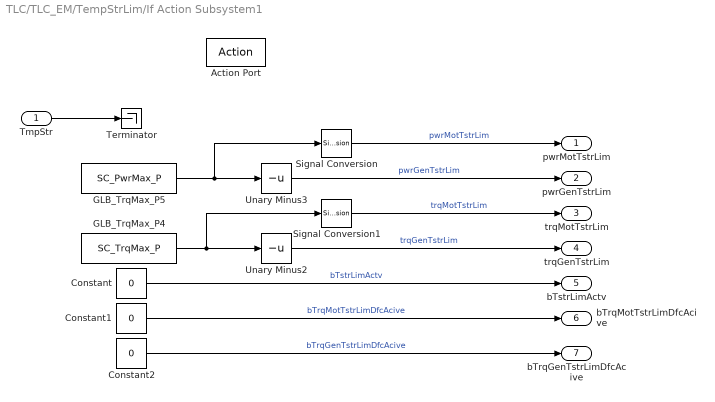
== system TLC/TLC_EM/TempStrLim/If Action Subsystem1 ==
  TmpStr : Inport
  Action Port : ActionPort  ActionPortLabel=else
  Constant : Constant  Value=0  OutDataTypeStr=boolean
  Constant1 : Constant  Value=0  OutDataTypeStr=boolean
  Constant2 : Constant  Value=0  OutDataTypeStr=boolean
  GLB_TrqMax_P4 : Constant  Value=SC_TrqMax_P  OutDataTypeStr=single
  GLB_TrqMax_P5 : Constant  Value=SC_PwrMax_P  OutDataTypeStr=single
  Signal Conversion : SignalConversion  OverrideOpt=off
  Signal Conversion1 : SignalConversion  OverrideOpt=off
  Terminator : Terminator
  Unary Minus2 : UnaryMinus
  Unary Minus3 : UnaryMinus
  pwrMotTstrLim : Outport  VectorParamsAs1DForOutWhenUnconnected=off
  pwrGenTstrLim : Outport  Port=2  VectorParamsAs1DForOutWhenUnconnected=off
  trqMotTstrLim : Outport  Port=3  VectorParamsAs1DForOutWhenUnconnected=off
  trqGenTstrLim : Outport  Port=4  VectorParamsAs1DForOutWhenUnconnected=off
  bTstrLimActv : Outport  Port=5  VectorParamsAs1DForOutWhenUnconnected=off
  bTrqMotTstrLimDfcAcive : Outport  Port=6  VectorParamsAs1DForOutWhenUnconnected=off
  bTrqGenTstrLimDfcAcive : Outport  Port=7  VectorParamsAs1DForOutWhenUnconnected=off
  wires:
  GLB_TrqMax_P4/1 -> Unary Minus2/1, Signal Conversion1/1
  GLB_TrqMax_P5/1 -> Unary Minus3/1, Signal Conversion/1
  Unary Minus2/1 -> trqGenTstrLim/1  "trqGenTstrLim"
  Unary Minus3/1 -> pwrGenTstrLim/1  "pwrGenTstrLim"
  TmpStr/1 -> Terminator/1
  Constant/1 -> bTstrLimActv/1  "bTstrLimActv"
  Constant1/1 -> bTrqMotTstrLimDfcAcive/1  "bTrqMotTstrLimDfcAcive"
  Constant2/1 -> bTrqGenTstrLimDfcAcive/1  "bTrqGenTstrLimDfcAcive"
  Signal Conversion/1 -> pwrMotTstrLim/1  "pwrMotTstrLim"
  Signal Conversion1/1 -> trqMotTstrLim/1  "trqMotTstrLim"

== matlab function TLC/TLC_EM/iDclinkLim/PID Controller ==
  data: Out output; error input; kpIdcMax input; kiIdcMax input
function Out = fcn(error,kpIdcMax,kiIdcMax)
%
persistent Temp;

if isempty(Temp)
    Temp = single(0);
end
    
Temp = kpIdcMax*kiIdcMax*error*single(0);
Out = Temp;
